simulink model "SimplePID"  (R2026a)
settings: Solver=VariableStepAuto
libraries: ros2lib x3
settings Model: Creator=hashaam1217  LastModifiedBy=hashaam1217

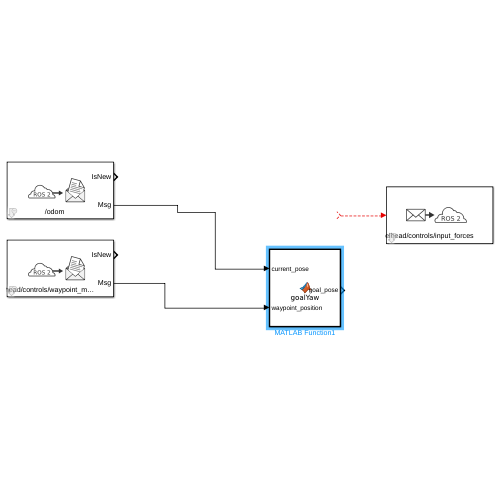
[thumbnail: Simulink's stored preview of the top-level diagram]
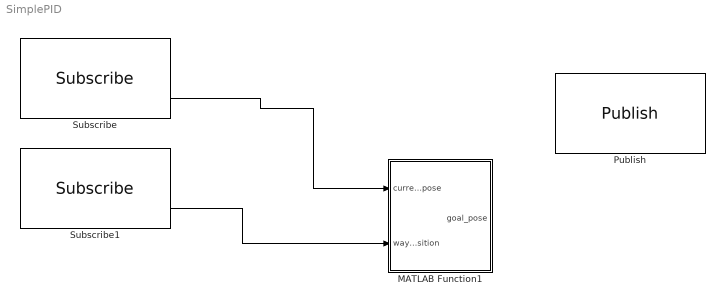
== system SimplePID ==
  MATLAB Function1 : MATLAB Function  TreatAsAtomicUnit=on
  Publish : ros2lib/Publish  topicSource=Select from ROS network  topic=/steelhead/controls/input_forces  messageType=geometry_msgs/Wrench  QOSHistory=Keep last  QOSDepth=10  QOSReliability=Reliable  QOSDurability=Volatile  QOSDeadline=Inf  QOSLifespan=Inf  QOSLiveliness=Automatic  QOSLeaseDuration=Inf  QOSAvoidROSNamespaceConventions=off
  Subscribe : ros2lib/Subscribe  topicSource=Select from ROS network  topic=/odom  messageType=nav_msgs/Odometry  sampleTime=0.02  QOSHistory=Keep all  QOSDepth=10  QOSReliability=Reliable  QOSDurability=Volatile  QOSDeadline=Inf  QOSLifespan=Inf  QOSLiveliness=Automatic  QOSLeaseDuration=Inf  QOSAvoidROSNamespaceConventions=off
  Subscribe1 : ros2lib/Subscribe  topicSource=Select from ROS network  topic=/steelhead/controls/waypoint_marker/current_goal  messageType=geometry_msgs/Point  sampleTime=-1  QOSHistory=Keep last  QOSDepth=10  QOSReliability=Reliable  QOSDurability=Volatile  QOSDeadline=Inf  QOSLifespan=Inf  QOSLiveliness=Automatic  QOSLeaseDuration=Inf  QOSAvoidROSNamespaceConventions=off
  wires:
  Subscribe/2 -> MATLAB Function1/1(current_pose)
  ? -> Publish/1
  Subscribe1/2 -> MATLAB Function1/2(waypoint_position)

== matlab function SimplePID/MATLAB Function1 ==
  data: current_pose input; goal_pose output; waypoint_position input
function goal_pose = goalYaw(current_pose, waypoint_position)
    current_position = current_pose.position; 
    current_orientation = current_pose.orientation;
    vector_x = waypoint_position.x - current_position.x;
    vector_y = waypoint_position.y - current_position.y;
    vector_z = waypoint_position.z - current_position.z;

    goal_pose.yaw = atan(vector_y, vector_x) - current_orientation;
    goal.pose.yaw = mod(goal_pose.yaw + pi, 2*pi) - pi;
    goal.pose.x   = vector_x;
    goal.pose.y   = vector_y;
    goal.pose.z   = vector_z;
end
